simulink model "DueSerbatoiProMaxSimulink"  (R2022b)
settings: Solver=VariableStepAuto  StartTime=0.0  StopTime=5000  RelTol=1e-3
values from neighbouring files (symbols this model uses):
  C1 = 500    [DueSerbatoiProMax.m]    (also in DueSerbatoiProMax_frequenza.m = 100; DueSerbatoiProMax_tempo.m = 100; SimulinkValues.m = 100)
  C2 = 120    [DueSerbatoiProMax.m]    (also in DueSerbatoiProMax_frequenza.m; DueSerbatoiProMax_tempo.m; SimulinkValues.m)
  g = 9.81    [DueSerbatoiProMax.m]    (also in DueSerbatoiProMax_frequenza.m; DueSerbatoiProMax_tempo.m; SimulinkValues.m)
  L1 = 1    [DueSerbatoiProMax.m]    (also in DueSerbatoiProMax_frequenza.m; DueSerbatoiProMax_tempo.m; SimulinkValues.m)
  Pa = 5    [DueSerbatoiProMax.m]    (also in DueSerbatoiProMax_tempo.m; SimulinkValues.m = 1)
  Q11 = 0    [SimulinkValues.m]
  Q12 = 5    [SimulinkValues.m]
  Q21 = 0    [SimulinkValues.m]
  Q22 = 4    [SimulinkValues.m]
  R1 = 1    [DueSerbatoiProMax.m]    (also in DueSerbatoiProMax_frequenza.m; DueSerbatoiProMax_tempo.m; SimulinkValues.m)
  R2 = 1    [DueSerbatoiProMax.m]    (also in DueSerbatoiProMax_frequenza.m; DueSerbatoiProMax_tempo.m; SimulinkValues.m)
  ro = 1000    [DueSerbatoiProMax.m]    (also in DueSerbatoiProMax_frequenza.m; DueSerbatoiProMax_tempo.m; SimulinkValues.m)
settings Model: Creator=giuli  LastModifiedBy=giuli

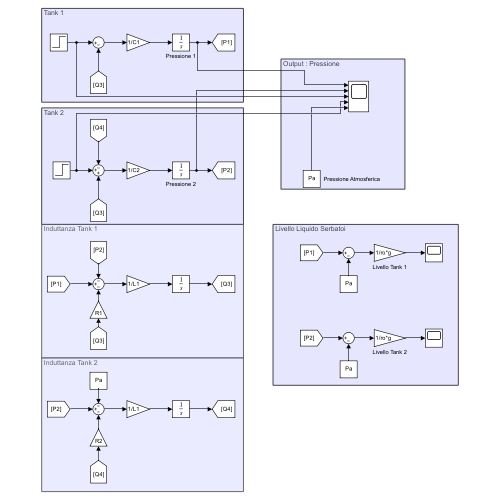
[thumbnail: Simulink's stored preview of the top-level diagram]
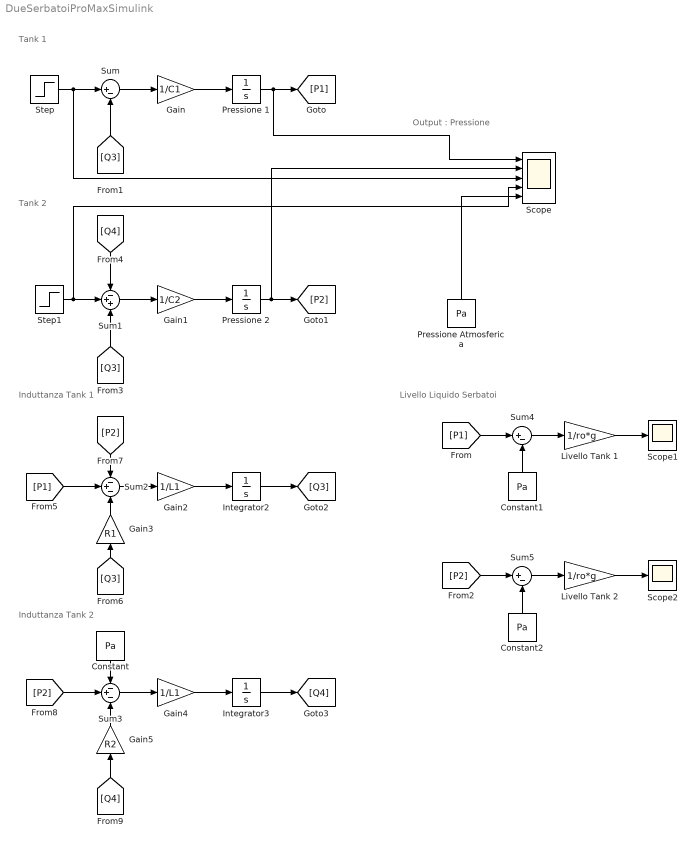
== system DueSerbatoiProMaxSimulink ==
  note: Livello Liquido Serbatoi
  note: Output : Pressione
  note: Induttanza Tank 2
  note: Induttanza Tank 1
  note: Tank 2
  note: Tank 1
  Constant : Constant  Value=Pa
  Constant1 : Constant  Value=Pa
  Constant2 : Constant  Value=Pa
  Gain : Gain  Gain=1/C1
  Gain1 : Gain  Gain=1/C2
  Gain2 : Gain  Gain=1/L1
  Gain3 : Gain  Gain=R1
  Gain4 : Gain  Gain=1/L1
  Gain5 : Gain  Gain=R2
  Integrator2 : Integrator
  Integrator3 : Integrator
  Livello Tank 1 : Gain  Gain=1/ro*g
  Livello Tank 2 : Gain  Gain=1/ro*g
  Pressione 1 : Integrator
  Pressione 2 : Integrator
  Pressione Atmosferica : Constant  Value=Pa
  Scope : Scope  NumInputPorts=5
  Scope1 : Scope
  Scope2 : Scope
  Step : Step  Time=1500  Before=Q11  After=Q12  SampleTime=0.1
  Step1 : Step  Time=3500  Before=Q21  After=Q22  SampleTime=0.1
  Sum : Sum  Inputs=|+-
  Sum1 : Sum  Inputs=-++
  Sum2 : Sum  Inputs=-+-
  Sum3 : Sum  Inputs=-+-
  Sum4 : Sum  Inputs=|+-
  Sum5 : Sum  Inputs=|+-
  wires:
  Gain/1 -> Pressione 1/1
  Sum/1 -> Gain/1
  Pressione 1/1 -> Scope/1, [P1]
  Step/1 -> Sum/1, Scope/3
  [Q3] -> Sum/2
  Pressione 2/1 -> Scope/2, [P2]
  Sum1/1 -> Gain1/1
  Gain1/1 -> Pressione 2/1
  Step1/1 -> Scope/4, Sum1/2
  [Q3] -> Sum1/3
  [Q4] -> Sum1/1
  [P2] -> Sum2/1
  [P1] -> Sum2/2
  Gain2/1 -> Integrator2/1
  Sum2/1 -> Gain2/1
  Integrator2/1 -> [Q3]
  Gain3/1 -> Sum2/3
  [Q3] -> Gain3/1
  [Q4] -> Gain5/1
  Gain5/1 -> Sum3/3
  Integrator3/1 -> [Q4]
  Sum3/1 -> Gain4/1
  Gain4/1 -> Integrator3/1
  [P2] -> Sum3/2
  Constant/1 -> Sum3/1
  Pressione Atmosferica/1 -> Scope/5
  [P1] -> Sum4/1
  Constant1/1 -> Sum4/2
  Sum4/1 -> Livello Tank 1/1
  Livello Tank 1/1 -> Scope1/1
  Livello Tank 2/1 -> Scope2/1
  Sum5/1 -> Livello Tank 2/1
  Constant2/1 -> Sum5/2
  [P2] -> Sum5/1
